simulink model "onetwo"  (R2014a)
settings: Solver=ode45  StartTime=0.0  StopTime=10.0  RelTol=1e-3
settings Model: Creator=trigg  LastModifiedBy=trigg

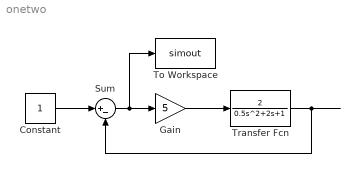
== system onetwo ==
  Constant : Constant
  Gain : Gain  Gain=5
  Sum : Sum  Inputs=|+-
  To Workspace : ToWorkspace  VariableName=simout  SaveFormat=Timeseries  SampleTime=-1
  Transfer Fcn : TransferFcn  Numerator=[2]  Denominator=[0.5 2 1]
  wires:
  Constant/1 -> Sum/1
  Sum/1 -> To Workspace/1, Gain/1
  Gain/1 -> Transfer Fcn/1
  Transfer Fcn/1 -> Sum/2
